simulink model "provaprova"  (R2024b)
settings: Solver=VariableStepAuto  StartTime=0.0  StopTime=10.0  RelTol=1e-3
values from neighbouring files (symbols this model uses):
  A = stabilita_AS(g, m)    [forwarding.m]    (also in stabilita_AS.m = [0, -g/m, 0)
  AA = A - B * K    [stabilita_AS.m]
  B = [0; 0; k]    [stabilita_AS.m]
  K = acker(A, B, desired_poles)    [stabilita_AS.m]
settings Model: Creator=Ilaria  LastModifiedBy=Ilaria

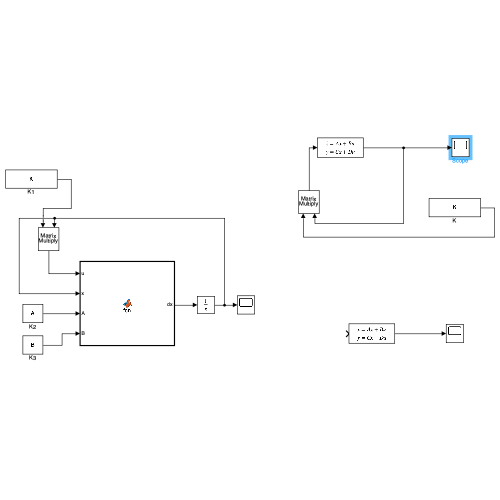
[thumbnail: Simulink's stored preview of the top-level diagram]
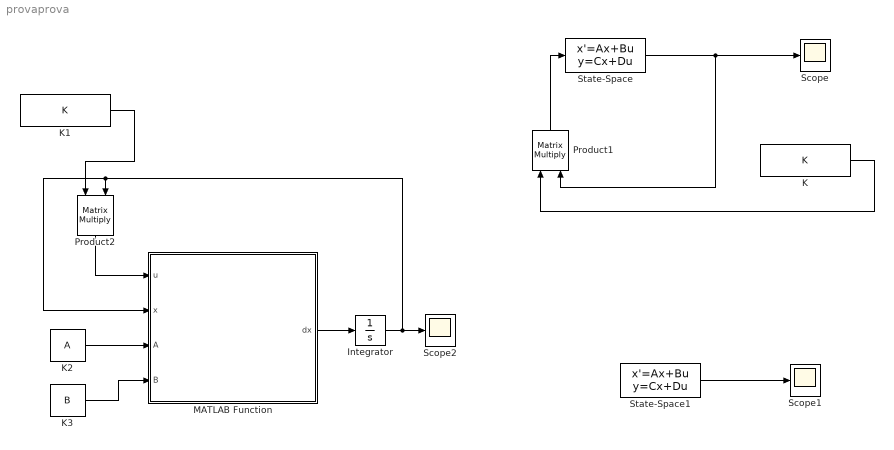
== system provaprova ==
  Integrator : Integrator
  K : Constant  Value=K  VectorParams1D=off
  K1 : Constant  Value=K  VectorParams1D=off
  K2 : Constant  Value=A  VectorParams1D=off
  K3 : Constant  Value=B  VectorParams1D=off
  MATLAB Function : MATLAB Function  TreatAsAtomicUnit=on
  Product1 : Product  Multiplication=Matrix(*)
  Product2 : Product  Multiplication=Matrix(*)
  Scope : Scope
  Scope1 : Scope
  Scope2 : Scope
  State-Space : StateSpace  A=A  B=B  C=eye(4)  D=[0; 0; 0; 0]  InitialCondition=[1,2,0,4]
  State-Space1 : StateSpace  A=AA  B=B  C=eye(4)  D=[0; 0; 0; 0]  InitialCondition=[1,2,0,4]
  wires:
  State-Space/1 -> Scope/1, Product1/2
  K/1 -> Product1/1
  Product1/1 -> State-Space/1
  State-Space1/1 -> Scope1/1
  MATLAB Function/1(dx) -> Integrator/1
  Integrator/1 -> MATLAB Function/2(x), Product2/2, Scope2/1
  K1/1 -> Product2/1
  Product2/1 -> MATLAB Function/1(u)
  K2/1 -> MATLAB Function/3(A)
  K3/1 -> MATLAB Function/4(B)

== matlab function provaprova/MATLAB Function ==
  data: u input; x input; dx output; A input; B input
function dx  = fcn(u, x, A,B)
    
    dx = A*x + B*u;
end
